simulink model "sedemo_async_stateflow_ent"  (Simulink 7.5)
settings: Solver=VariableStepDiscrete  StartTime=0.0  StopTime=30  MaxStep=inf  RelTol=1e-3
libraries: simeventsgenerators1 x2, simulink x2, simeventstranslate1 x1, simeventssink1 x1, simeventsrouting1 x1, simeventsattributes2 x1, simeventsserver1 x1, simeventsinfo x1
settings Model: Creator=The MathWorks Inc.
settings DataIOCC: SaveOutput=off  SaveTime=off
settings OptimizationCC: InitFltsAndDblsToZero=on  EfficientMapNaN2IntZero=off
settings DebuggingCC: AlgebraicLoopMsg=error  SaveWithParameterizedLinksMsg=none  SignalResolutionControl=TryResolveAllWithWarning  SolverPrmCheckMsg=none  StrictBusMsg=Warning
settings GRTTargetCC: TargetFcnLib=ansi_tfl_tmw.mat
settings SimEventsCC: propDiagAttribOutput=1  propDiagFcnCallOutput=1  propDiagStatOutput=0

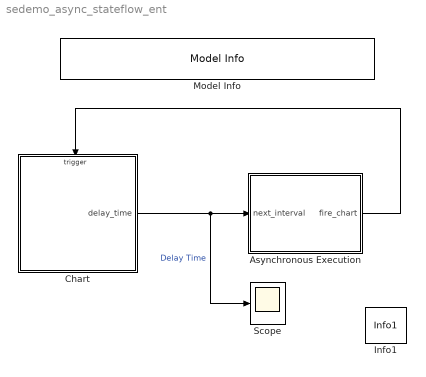
== system sedemo_async_stateflow_ent ==
  Asynchronous Execution : Subsystem
  Chart : Stateflow chart  TreatAsAtomicUnit=on
      settings: PropExecContextOutsideSubsystem=on
  Info1 : simeventsinfo/Info1  SystemSampleTime=-1  file_name=sedemo_async_stateflow
  Model Info : simulink/Model-Wide Utilities/Model Info  SystemSampleTime=-1  InitialBlockCM=None  BlockCM=None  Frame=off  DisplayStringWithTags=|  HorizontalTextAlignment=Center  LeftAlignmentValue=0.5  SourceBlockDiagram=sedemo_async_stateflow_ent  TagMaxNumber=20
      | Asynchronous Execution of a
      | Stateflow Chart (using Entities)
  Scope : Scope
      settings: TickLabels=on  TimeRange=30  YMin=0  YMax=10
  wires:
  Chart/1(delay_time) -> Asynchronous Execution/1(next_interval), Scope/1  "Delay Time"
  Asynchronous Execution/1(fire_chart) -> Chart/Trigger

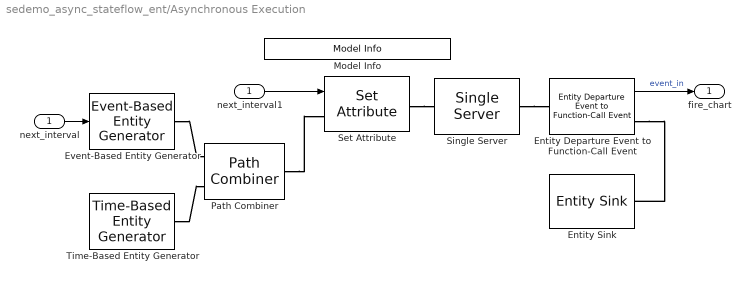
== system sedemo_async_stateflow_ent/Asynchronous Execution ==
  next_interval : Inport
  Entity Departure Event to Function-Call Event : simeventstranslate1/Entity Departure Event to Function-Call Event  Priority=1  SystemSampleTime=-1  TimingFunctionCallF1=After entity departure  EnableE1Port=off  EnableF2Port=off  TimingFunctionCallF2=Before entity departure  EnableE2Port=off  StatNumberDeparted=Off  StatNumberF1Calls=Off  StatNumberF2Calls=Off  IsInsideAFB=off
  Entity Sink : simeventssink1/Entity Sink  Priority=1  SystemSampleTime=-1  AvailableForArrivals=on  StatNumberArrived=Off
  Event-Based Entity Generator : simeventsgenerators1/Entity Generators/Event-Based Entity Generator  Priority=1  DialogController=des_ddg_create  DialogControllerArgs=DataTag3  SystemSampleTime=-1  GenerateEntitiesUpon=Sample time hit from port ts  SignalEdgeType=Either  SpecifyEventPriority=on  PriorityEntityGeneration=600  GenerateEntityAtSimulationStart=on  AllowBlocking=on  ResponseDuringBlockage=Discard generated entities  EntityType=Blank  StatNumberDeparted=Off  StatPendingEntity=Off  StatAverageIntergenerationTime=Off
  Model Info : simulink/Model-Wide Utilities/Model Info  SystemSampleTime=-1  InitialBlockCM=None  BlockCM=None  Frame=off  DisplayStringWithTags=Delayed Entities  HorizontalTextAlignment=Center  LeftAlignmentValue=0.5  SourceBlockDiagram=sedemo_delayed_stateflow_ent  TagMaxNumber=20
  Path Combiner : simeventsrouting1/Path Combiner  Priority=1  SystemSampleTime=-1  NumberInputPorts=2  InputPortPrecedence=IN1 port  InitialSeed=45675  SpecifyEventPriority=off  PriorityPathCombinerPortPrecedenceSelection=4100  StatNumberDeparted=Off  StatLastArrivalPort=Off  EvaluatedNumPorts=2
  Set Attribute : simeventsattributes2/Set Attribute  Priority=1  DialogController=des_ddg_create  DialogControllerArgs=DataTag6  SystemSampleTime=-1  AttributeFrom=Signal port  AttributeName=DelayTime  AttributeTreatAsVector=1  AttributeValue=1  AttributeCreate=on  StatNumberDeparted=Off  EvaluatedAttributeValue={[]}
  Single Server : simeventsserver1/Single Server  Priority=1  SystemSampleTime=-1  ServiceTimeFrom=Attribute  ServiceTime=1  AttributeName=DelayTime  PriorityServiceCompletion=500  PermitPreemption=off  SortingAttributeName=PriorityAttributeName  SortingDirection=Ascending  WriteToAttribute=off  ResidualAttributeName=ResidualServiceTime  CreateAttribute=on  EnableTOPort=off  StatNumberDeparted=Off  StatNumberInBlock=Off  StatNumberPreempted=Off  StatPendingEntity=Off  StatAverageWait=Off  StatUtilization=Off  StatNumberTimedout=Off
  Time-Based Entity Generator : simeventsgenerators1/Entity Generators/Time-Based Entity Generator  Priority=1  DialogController=des_ddg_create  DialogControllerArgs=DataTag9  SystemSampleTime=-1  GenerateEntitiesUpon=Intergeneration time from dialog  Distribution=Constant  Minimum=0  Maximum=1  Mean=1  InitialSeed=12345  Period=inf  PriorityEntityGeneration=300  GenerateEntityAtSimulationStart=on  ResponseWhenBlocked=Pause generation  ResponseWhenUnblocked=Immediate restart  EntityType=Blank  StatNumberDeparted=Off  StatPendingEntity=Off  StatAverageIntergenerationTime=Off
  next_interval1 : InportShadow  Port=1
  fire_chart : Outport
  wires:
  Entity Departure Event to Function-Call Event/1 -> fire_chart/1  "event_in"
  next_interval1/1 -> Set Attribute/1
  next_interval/1 -> Event-Based Entity Generator/1
  connections:
  Set Attribute/RConn1 -- Single Server/LConn1
  Single Server/RConn1 -- Entity Departure Event to Function-Call Event/LConn1
  Entity Departure Event to Function-Call Event/RConn1 -- Entity Sink/LConn1
  Event-Based Entity Generator/RConn1 -- Path Combiner/LConn1
  Time-Based Entity Generator/RConn1 -- Path Combiner/LConn2
  Path Combiner/RConn1 -- Set Attribute/LConn1

== stateflow chart Chart ==
  settings: sampleTime=1
  state Active
    entry:delay_time = delay_time + 1;
  state End
  note: Stateflow Chart Logic
  Active -> End [order 1] : [delay_time > 5]
  (default) -> Active : {delay_time=0;}
  Active -> Active [order 2] : event_in
  data: delay_time output double
  events: event_in input FUNCTION_CALL_EVENT
